simulink model "BC_MR"  (R2025b)
settings: Solver=FixedStepAuto  StartTime=0.0  StopTime=15  FixedStep=TsELEC  RelTol=1e-3  EnableMultiTasking=on
InitFcn:
  | TsELEC = Ts;
  | TsMECH = 5e-4;
  | TsTHERMAL = 1e-3;
  | 
  | Ts_speed = 1e-4;
  | Ts_inverter = Ts;
  | Ts_motor = Ts;
  | Ts_simulink = Ts;
  | 
  | 
  | PM = 0.03*10; % Permanent magnet flux linkage
  | Ld = 2e-3;  % d-axis inductance
  | Lq = 2e-3;  % q-axis inductance
  | L0 = 2e-3;  % 0-axis inductance
  | Rs = 0.0013; % Stator resistance
  | N = 2; % Number of pole pairs
  | J = 0.2; % Moment of inertia
values from neighbouring files (symbols this model uses):
  combustor_volume = 0.001    [initParams.mat]
  compressor =     [initParams.mat]
  flow_area = 0.002    [initParams.mat]
  scale_factor = 5    [initParams.mat]
  Ts = 5e-05    [initParams.mat]
  turbine =     [initParams.mat]
undefined symbols (not defined in the file or in its folder): DiscIntNeverNeededParam
libraries: fl_lib x42, nesl_utility x16, BraytonCycle_lib x4
(part 1 of 4)
settings Model: Creator=gdudgeon  LastModifiedBy=gdudgeon
settings SolverCC: ConcurrentTasks=on  AlgebraicLoopSolver=TrustRegion  PositivePriorityOrder=on  AutoInsertRateTranBlk=on
settings DataIOCC: SaveFormat=StructureWithTime
settings OptimizationCC: BlockReduction=off  OptimizeBlockIOStorage=off
settings DebuggingCC: TasksWithSamePriorityMsg=none  UnconnectedInputMsg=warning  UnconnectedOutputMsg=warning  UnconnectedLineMsg=warning
settings HardwareCC: ProdBitPerLong=64.0  ProdLongLongMode=on  ProdHWDeviceType=Intel->x86-64 (Linux 64)
settings ModelReferenceCC: EnableRefExpFcnMdlSchedulingChecks=on  ModelReferenceNumInstancesAllowed=Single
settings RTWCC: SystemTargetFile=speedgoat.tlc  TemplateMakefile=slrealtime_default_tmf  Toolchain=Simulink Real-Time Toolchain  BuildConfiguration=Faster Runs  CodeExecutionProfiling=on  TargetLang=C++  GPUComputeCapability=3.5  Description=Speedgoat Real-Time Target Machine
settings SimulinkRealTimeTargetCC: SLRTFileLogMaxRuns=1.0  ExtModeMaxTrigDuration=10.0  ExtModeStaticAllocSize=1000000.0  ExtModeTransport=0.0  MultiwordLength=2048.0  DynamicStringBufferSize=256.0  PreserveMATLABNamespacesInGeneratedCode=on  SubcomponentCodeInterfacePackaging=Nonreusable function  MATLABClassNameForMDSCustomization=Simulink.SoftwareTarget.GRTCustomization  InstructionSetFMA=off  LogToMDFFile=off

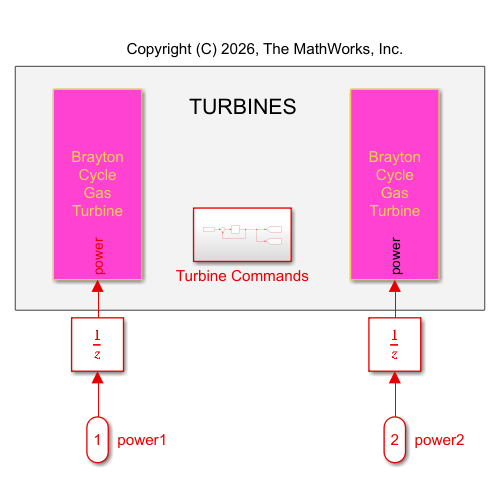
[thumbnail: Simulink's stored preview of the top-level diagram]
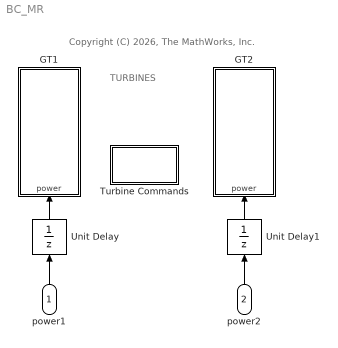
== system BC_MR ==
  note: Copyright (C) 2026, The MathWorks, Inc.
  note: TURBINES
  power1 : Inport
  power2 : Inport  Port=2
  GT1 : Subsystem
      settings: PortSchema="{\"entries\":[{\"content\":{\"sides\":[{\"content\":{\"connectorIds\":[]},\"type\":\"ConnectorPlacement.EquallySpacedRectSide\",\"uuid\":\"a04ed74d-c3e9-4f62-bdbe-b0696cf0a26f\"},{\"content\":{\"connectorIds\":[\"In1\"],\"side\":\"RIGHT\"},\"type\":\"ConnectorPlacement.EquallySpacedRectSide\",\"uuid\":\"20b35612-2c43-4c02-89ae-fd47f8e8a57e\"},{\"content\":{\"connectorIds\":[],\"side\":\"TOP\"},\"type\":\"ConnectorPlacement.EquallySpacedRectSide\",\"uuid\":\"6f0a7e20-92d8-4aae-b92c-6e7431fc1b6b\"}]},\"type\":\"ConnectorPlacement.EquallySpacedConnector\",\"uuid\":\"8c9a37df-85b6-4aaf-ab49-91d007aa59bf\"}],\"packageUris\":[\"http://schema.mathworks.com/mf0/Connector/19700101\"],\"version\":\"1.0\"}"
      mask Display: disp('Brayton\nCycle\nGas\nTurbine')
  GT2 : Subsystem
      settings: PortSchema="{\"entries\":[{\"content\":{\"sides\":[{\"content\":{\"connectorIds\":[]},\"type\":\"ConnectorPlacement.EquallySpacedRectSide\",\"uuid\":\"d41540ca-81a6-46f6-a39a-240134fd70c4\"},{\"content\":{\"connectorIds\":[\"In1\"],\"side\":\"RIGHT\"},\"type\":\"ConnectorPlacement.EquallySpacedRectSide\",\"uuid\":\"a1ae4ce1-21e7-4c30-9d08-a3be7360a772\"},{\"content\":{\"connectorIds\":[],\"side\":\"TOP\"},\"type\":\"ConnectorPlacement.EquallySpacedRectSide\",\"uuid\":\"66800067-f51d-4599-9d24-34a547b1a44f\"}]},\"type\":\"ConnectorPlacement.EquallySpacedConnector\",\"uuid\":\"ebdf8939-58d4-4b69-bce0-e05b52e5db49\"}],\"packageUris\":[\"http://schema.mathworks.com/mf0/Connector/19700101\"],\"version\":\"1.0\"}"
      mask Display: disp('Brayton\nCycle\nGas\nTurbine')
  Turbine Commands : Subsystem
  Unit Delay : UnitDelay  SampleTime=TsELEC  HasFrameUpgradeWarning=on
  Unit Delay1 : UnitDelay  SampleTime=TsELEC  HasFrameUpgradeWarning=on
  wires:
  power1/1 -> Unit Delay/1
  power2/1 -> Unit Delay1/1
  Unit Delay/1 -> GT1/1(power)
  Unit Delay1/1 -> GT2/1(power)
